simulink model "flightSim"  (R2023a)
settings: Solver=ode45  StartTime=0.0  StopTime=350  RelTol=1e-3
values from neighbouring files (symbols this model uses):
  g = 9.81    [parameters.m]
  gam_0 = pi/2    (= 1.57079632679)    [parameters.m]
  gam_in = 0.10    (= 0.1)    [parameters.m]
  h_0 = 0    [parameters.m]
  m_dot = 132.46    [parameters.m]
  m_zfw = m_pay + m_dry    (= 6360.7)    [parameters.m]
  PID_Gain = d_2/J_y    (= 0.025)    [parameters.m]
  R_E = 6371e3    (= 6371000)    [parameters.m]
  t_turn = 30.0    (= 30)    [parameters.m]
  v_0 = 0.01    [parameters.m]
libraries: slpidlib x1, simulink x1
settings Model: Creator=Administrator  LastModifiedBy=Administrator

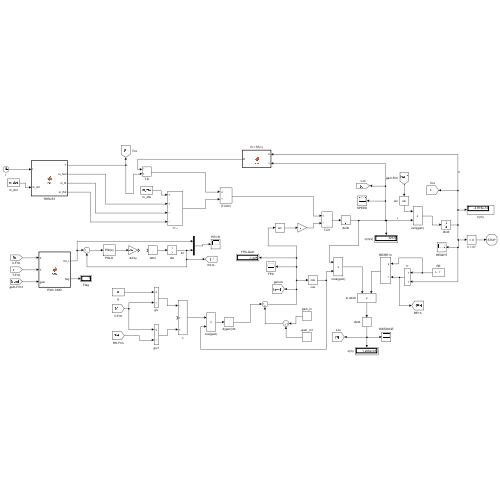
[thumbnail: Simulink's stored preview of the top-level diagram]
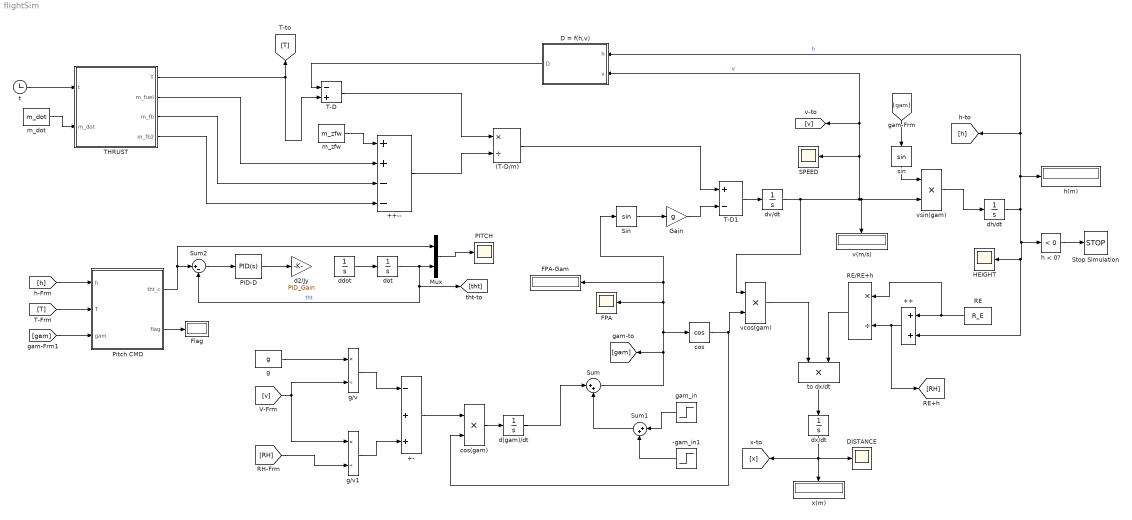
== system flightSim ==
  (T-D/m) : Product  Inputs=*/
  ++ : Sum
  ++-- : Sum  Inputs=++--
  +- : Sum  Inputs=-++
  -gam_in1 : Step  Time=t_turn+1  Before=-gam_in  After=-gam_in  SampleTime=0
  D = f(h,v) : MATLAB Function  TreatAsAtomicUnit=on
  DISTANCE : Scope
  FPA : Scope
  FPA-Gam : Display
  Flag : Display
  Gain : Gain  Gain=g
  HEIGHT : Scope
  Mux : Mux  Inputs=2
  PID-D : slpidlib/PID Controller  Controller=PID  Form=Parallel  TimeDomain=Continuous-time  UseExternalTs=off  SampleTime=-1  IntegratorMethod=Forward Euler  FilterMethod=Forward Euler  ControllerParametersSource=internal  P=0  I=0  UseKiTs=off  D=200/5  N=100  UseFilter=on  TunerSelectOption=Transfer Function Based (PID Tuner App)  InitialConditionSource=internal  InitialConditionForIntegrator=0  InitialConditionForFilter=0  DifferentiatorICPrevScaledInput=0  ExternalReset=none  TrackingMode=off  Kt=1  LimitOutput=off  SatLimitsSource=internal  UpperSaturationLimit=inf  LowerSaturationLimit=-inf  LinearizeAsGain=on  AntiWindupMode=none  Kb=1  LimitIntegrator=off  UpperIntegratorSaturationLimit=inf  LowerIntegratorSaturationLimit=-inf  POutMin=[]  POutMax=[]  IOutMin=[]  IOutMax=[]  DOutMin=[]  DOutMax=[]  NOutMin=[]  NOutMax=[]  SumOutMin=[]  SumOutMax=[]  SaturationOutMin=[]  SaturationOutMax=[]  PParamMin=[]  PParamMax=[]  IParamMin=[]  IParamMax=[]  DParamMin=[]  DParamMax=[]  NParamMin=[]  NParamMax=[]  KbParamMin=[]  KbParamMax=[]  KtParamMin=[]  KtParamMax=[]  KbOutMin=[]  KbOutMax=[]  KtOutMin=[]  KtOutMax=[]  IntegratorOutMin=[]  IntegratorOutMax=[]  FilterOutMin=[]  FilterOutMax=[]  SumI1OutMin=[]  SumI1OutMax=[]  SumI2OutMin=[]  SumI2OutMax=[]  SumI3OutMin=[]  SumI3OutMax=[]  SumI4OutMin=[]  SumI4OutMax=[]  SumDOutMin=[]  SumDOutMax=[]  DifferentiatorOutMin=[]  DifferentiatorOutMax=[]  FilterDiffOutCoefMin=[]  FilterDiffOutCoefMax=[]  ReciprocalOutMin=[]  ReciprocalOutMax=[]  SumDenOutMin=[]  SumDenOutMax=[]  SumNumOutMin=[]  SumNumOutMax=[]  DivideOutMin=[]  DivideOutMax=[]  UdiffTsProdOutMin=[]  UdiffTsProdOutMax=[]  NTsProdOutMin=[]  NTsProdOutMax=[]  UintegralTsProdOutMin=[]  UintegralTsProdOutMax=[]  UngainTsProdOutMin=[]  UngainTsProdOutMax=[]  ClampingZeroOutDataTypeStr=Inherit: Inherit via back propagation  ClampingZeroOutMin=[]  ClampingZeroOutMax=[]  FilterDenConstantOutDataTypeStr=Inherit: Inherit via back propagation  FilterDenConstantOutMin=[]  FilterDenConstantOutMax=[]  PCopyOutDataTypeStr=Inherit: Inherit via back propagation  PCopyOutMin=[]  PCopyOutMax=[]  NCopyOutDataTypeStr=Inherit: Inherit via back propagation  NCopyOutMin=[]  NCopyOutMax=[]  IntegratorContinuousStateAttributes=''  IntegratorStateMustResolveToSignalObject=off  IntegratorRTWStateStorageClass=Auto  FilterContinuousStateAttributes=''  FilterStateMustResolveToSignalObject=off  FilterRTWStateStorageClass=Auto  ParallelPVariant=InternalParameters  IdealPVariant=Disabled  IVariant=InternalParameters  DVariant=InternalParameters  IntegratorVariant=Continuous  SatVariant=Disabled  AWVariant=Passthrough  PCopyVariant=Disabled  TRVariant=Disabled  FdbkBlocksVariant=Forward  IdealPFdbkVariant=Disabled  SatFdbkVariant=Disabled  DerivativeFilterVariant=ContFilter  NVariant=InternalParameters  NCopyVariant=Disabled  FilterICVariant=InternalICsFilter  IntegratorICVariant=InternalICs  ExternalResetVariant=Disabled  TRSumVariant=Passthrough  SumFdbkVariant=Disabled  SumVariant=Sum_PID  TsampFilterVariant=InternalTs  TsampNgainVariant=Passthrough  TsampIntegralVariant=Disabled_SignalSpec  ExternalSaturationOutDataTypeStr=Inherit: Same as second input
  PITCH : Scope
  Pitch CMD : MATLAB Function  TreatAsAtomicUnit=on
  RE : Constant  Value=R_E
  RE/RE+h : Product  Inputs=*/
  SPEED : Scope
  Sin : Trigonometry
  Stop Simulation : Stop
  Sum : Sum  Inputs=|++
  Sum1 : Sum  Inputs=|++
  Sum2 : Sum  Inputs=|+-
  T-D : Sum  Inputs=-+
  T-D1 : Sum  Inputs=+-
  THRUST : MATLAB Function  TreatAsAtomicUnit=on
  cos : Trigonometry  Operator=cos
  cos(gam) : Product
  d(gam)/dt : Integrator  InitialCondition=gam_0
  d2/Jy : Gain  Gain=PID_Gain
  ddot : Integrator  InitialCondition=gam_0
  dh/dt : Integrator  InitialCondition=h_0
  dot : Integrator  InitialCondition=gam_0
  dv/dt : Integrator  InitialCondition=v_0
  dx/dt : Integrator  InitialCondition=h_0
  g : Constant  Value=g
  g/v : Product  Inputs=*/
  g/v1 : Product  Inputs=*/
  gam_in : Step  Time=t_turn  Before=gam_in  After=0  SampleTime=0
  h < 0? : simulink/Logic and Bit Operations/Compare To Zero  relop=<  OutDataTypeStr=boolean
  h(m) : Display
  m_dot : Constant  Value=m_dot
  m_zfw : Constant  Value=m_zfw
  sin : Trigonometry
  t : Clock
  to dx/dt : Product
  v(m/s) : Display
  vcos(gam) : Product
  vsin(gam) : Product
  x(m) : Display
  wires:
  t/1 -> THRUST/1(t)
  m_dot/1 -> THRUST/2(m_dot)
  THRUST/1(T) -> T-D/2, [T]
  m_zfw/1 -> ++--/1
  THRUST/2(m_fuel) -> ++--/2
  THRUST/3(m_fb) -> ++--/3
  THRUST/4(m_fb2) -> ++--/4
  T-D/1 -> (T-D/m)/1
  ++--/1 -> (T-D/m)/2
  Sin/1 -> Gain/1
  Gain/1 -> T-D1/2
  (T-D/m)/1 -> T-D1/1
  T-D1/1 -> dv/dt/1
  dv/dt/1 -> vcos(gam)/1, vsin(gam)/2, v(m/s)/1, SPEED/1, D = f(h,v)/2(v), [v]  "v"
  vsin(gam)/1 -> dh/dt/1
  dh/dt/1 -> ++/2, HEIGHT/1, h < 0?/1, [h], D = f(h,v)/1(h), h(m)/1  "h"
  h < 0?/1 -> Stop Simulation/1
  D = f(h,v)/1(D) -> T-D/1
  RE/1 -> RE/RE+h/1, ++/1
  ++/1 -> [RH], RE/RE+h/2
  RE/RE+h/1 -> to dx/dt/2
  to dx/dt/1 -> dx/dt/1
  dx/dt/1 -> DISTANCE/1, [x], x(m)/1
  g/1 -> g/v/1
  [v] -> g/v1/1, g/v/2
  [RH] -> g/v1/2
  g/v1/1 -> +-/3
  g/v/1 -> +-/1
  +-/1 -> cos(gam)/1
  cos(gam)/1 -> d(gam)/dt/1
  d(gam)/dt/1 -> Sum/1
  Sum/1 -> FPA-Gam/1, Sin/1, FPA/1, cos/1, [gam]
  cos/1 -> cos(gam)/2, vcos(gam)/2
  vcos(gam)/1 -> to dx/dt/1
  [gam] -> sin/1
  sin/1 -> vsin(gam)/1
  Sum1/1 -> Sum/2
  gam_in/1 -> Sum1/1
  -gam_in1/1 -> Sum1/2
  [h] -> Pitch CMD/1(h)
  [T] -> Pitch CMD/2(T)
  [gam] -> Pitch CMD/3(gam)
  Pitch CMD/2(flag) -> Flag/1
  Pitch CMD/1(tht_c) -> Mux/1, Sum2/1
  Sum2/1 -> PID-D/1
  PID-D/1 -> d2/Jy/1
  ddot/1 -> dot/1
  dot/1 -> [tht], Sum2/2, Mux/2  "tht"
  Mux/1 -> PITCH/1

== matlab function flightSim/Pitch CMD ==
  settings: updateMethod=DISCRETE
  data: h input; tht_c output; T input; gam input; flag output
function [tht_c, flag] = fcn(h, T, gam)
% Code Generation

persistent f
persistent t_c

if isempty(f)
    f = 0;
end

if T <=0
    t_c = gam+pi;
    if t_c > pi
        t_c = pi;
    end
    f = 1;
elseif T <= 0 && h < 1000
    t_c = pi/2;
else
    t_c = gam;
end

flag = f;
tht_c = t_c;

== matlab function flightSim/THRUST ==
  settings: updateMethod=DISCRETE
  data: t input; T output; m_fuel output; m_fb output; m_fb2 output; m_dot input
function [T, m_fuel, m_fb, m_fb2] = fcn(t, m_dot)
% Codegeneration

persistent mfb
persistent mfb2

if isempty(mfb)
    mfb = 0;
end

if isempty(mfb2)
    mfb2 = 0;
end

mfuel = 21491.26;

if mfb <= 0.65*mfuel
    THR = 346961.2;
    mfb = t*m_dot;
else
    THR = 0;
end


if (125<t) && (t < 295)
    THR = -110000;
    mfb2 = (t - 125)*(m_dot/3)
end

T = THR;
m_fb = mfb;
m_fb2 = mfb2
m_fuel = mfuel;

== matlab function flightSim/D = f(h,v) ==
  data: h input; D output; v input
function D = fcn(h, v)
% Code Generation

CD = 0.075;     %Drag Coefficient
Di = 1.5;
A = pi * Di^2/4;

%Density ISA Model from NASA website
%# Troposphere
if h <= 11000
    T = 15.04 - 0.00649*h;
    p = 101.29 * ((T+273.1)/288.08)^5.258;
%Lower Stratosphere
elseif (11000 < h) && (h <+ 25000)
    T = -56.46;
    p = 22.65 * exp(1.73-0.000157*h);
else
    T = -131.21 + 0.00299*h;
    p = 2.488 * ((T+273.1)/216.6)^-11.388;
end

rho = p/(0.2896 * (T+273.1))

% drag force D
Drag = 0.5*rho*v^2*A*CD;

D = Drag;
